simulink model "LIMITATIONS"  (R2024b)
settings: configuration reference "STM32H7_Config" (kept outside this file)
settings Model: DataDictionary=Master_Dictionary.sldd  EnableAccessToBaseWorkspace=off  Creator=torni  LastModifiedBy=William
settings ConfigSetRef: SourceName=STM32H7_Config

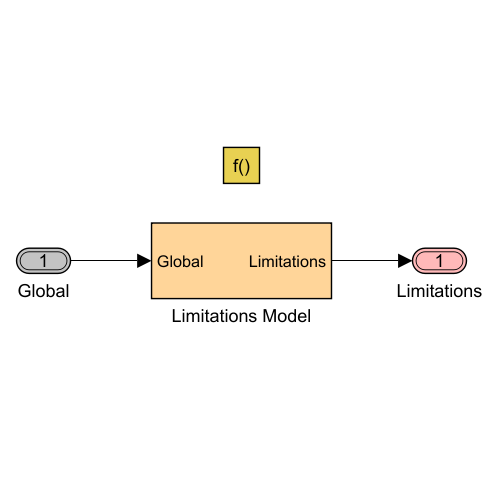
[thumbnail: Simulink's stored preview of the top-level diagram]
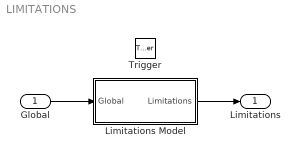
== system LIMITATIONS ==
  "Global " : Inport  OutDataTypeStr=Bus: Global
  Trigger : TriggerPort  TriggerType=function-call  VariantControl=Variant  PortDimensions=1
  "Limitations Model " : Subsystem
  Limitations : Outport  OutDataTypeStr=Bus: LimitationsBus  VectorParamsAs1DForOutWhenUnconnected=off
  wires:
  "Global "/1 -> "Limitations Model "/1(Global)
  "Limitations Model "/1(Limitations) -> Limitations/1

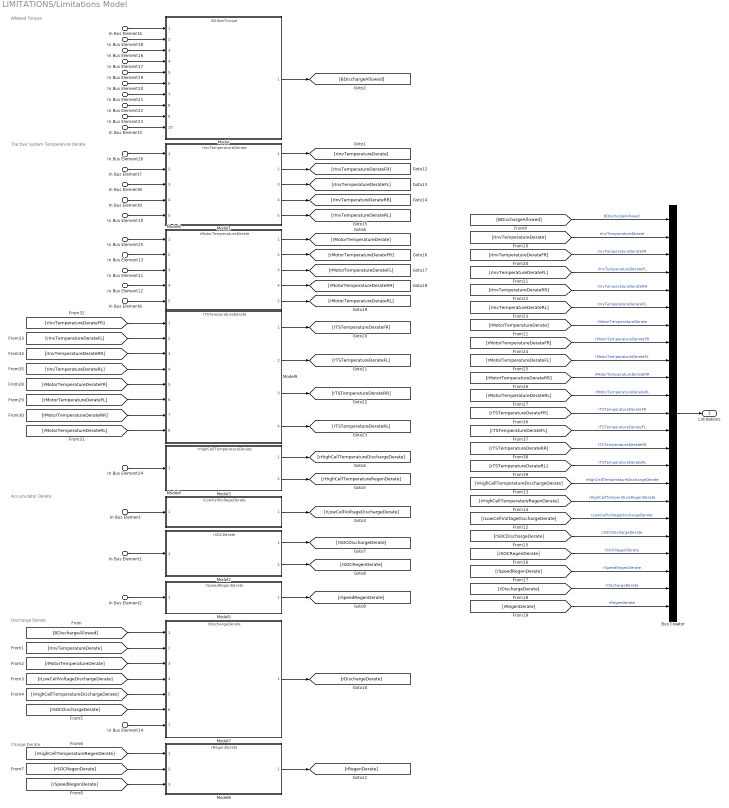
== system LIMITATIONS/Limitations Model  ==
  note: Allowed Torque
  note: Discharge Derate
  note: Charge Derate
  note: Tractive System Temperature Derate
  note: Accumulator Derate
  In Bus Element4 : Inport  PortName=Global  Element=StateflowBus.BReadyToDrive
  In Bus Element16 : Inport  PortName=Global  Element=SystemsBus.BThrottleError
  In Bus Element17 : Inport  PortName=Global  Element=SystemsBus.BBrakeError
  In Bus Element18 : Inport  PortName=Global  Element=SystemsBus.BBrakeOn
  In Bus Element19 : Inport  PortName=Global  Element=SystemsBus.BAppsOK
  In Bus Element25 : Inport  PortName=Global  Element=SystemsBus.TMotorMax
  In Bus Element26 : Inport  PortName=Global  Element=SystemsBus.TInvMax
  In Bus Element2 : Inport  PortName=Global  Element=SystemsBus.vChassis
  In Bus Element14 : Inport  PortName=Global  Element=SystemsBus.BEMSActivated
  In Bus Element20 : Inport  PortName=Global  Element=InverterSignalsBus.InverterFLSignalsBus.nMotorFL
  In Bus Element8 : Inport  PortName=Global  Element=InverterSignalsBus.InverterFLSignalsBus.TInvFL
  In Bus Element11 : Inport  PortName=Global  Element=InverterSignalsBus.InverterFLSignalsBus.TMotorFL
  In Bus Element21 : Inport  PortName=Global  Element=InverterSignalsBus.InverterFRSignalsBus.nMotorFR
  In Bus Element7 : Inport  PortName=Global  Element=InverterSignalsBus.InverterFRSignalsBus.TInvFR
  In Bus Element13 : Inport  PortName=Global  Element=InverterSignalsBus.InverterFRSignalsBus.TMotorFR
  In Bus Element22 : Inport  PortName=Global  Element=InverterSignalsBus.InverterRLSignalsBus.nMotorRL
  In Bus Element10 : Inport  PortName=Global  Element=InverterSignalsBus.InverterRLSignalsBus.TInvRL
  In Bus Element6 : Inport  PortName=Global  Element=InverterSignalsBus.InverterRLSignalsBus.TMotorRL
  In Bus Element23 : Inport  PortName=Global  Element=InverterSignalsBus.InverterRRSignalsBus.nMotorRR
  In Bus Element9 : Inport  PortName=Global  Element=InverterSignalsBus.InverterRRSignalsBus.TInvRR
  In Bus Element12 : Inport  PortName=Global  Element=InverterSignalsBus.InverterRRSignalsBus.TMotorRR
  In Bus Element24 : Inport  PortName=Global  Element=BMSSignalsBus.TCellMax
  In Bus Element : Inport  PortName=Global  Element=BMSSignalsBus.VCellMin
  In Bus Element1 : Inport  PortName=Global  Element=BMSSignalsBus.VDCAccumulator
  In Bus Element3 : Inport  PortName=Global  Element=BMSSignalsBus.IIVTS
  Bus Creator : BusCreator  Inputs=23  OutDataTypeStr=Bus: LimitationsBus
  Model : ModelReference  ModelNameDialog=BAllowTorque  SimulationMode=Normal  ModelReferenceVersion=13.6
  Model1 : ModelReference  ModelNameDialog=rInvTemperatureDerate.slx  SimulationMode=Normal  ModelReferenceVersion=13.6
  Model2 : ModelReference  ModelNameDialog=rSOCDerate.slx  SimulationMode=Normal  ModelReferenceVersion=13.6
  Model3 : ModelReference  ModelNameDialog=rHighCellTemperatureDerate.slx  SimulationMode=Normal  ModelReferenceVersion=13.6
  Model4 : ModelReference  ModelNameDialog=rLowCellVoltageDerate.slx  SimulationMode=Normal  ModelReferenceVersion=13.6
  Model5 : ModelReference  ModelNameDialog=rSpeedRegenDerate.slx  SimulationMode=Normal  ModelReferenceVersion=13.6
  Model6 : ModelReference  ModelNameDialog=rMotorTemperatureDerate.slx  SimulationMode=Normal  ModelReferenceVersion=13.6
  Model7 : ModelReference  ModelNameDialog=rDischargeDerate.slx  SimulationMode=Normal  ModelReferenceVersion=13.5
  Model8 : ModelReference  ModelNameDialog=rRegenDerate.slx  SimulationMode=Normal  ModelReferenceVersion=13.5
  Model9 : ModelReference  ModelNameDialog=rTSTemperatureDerate.slx  SimulationMode=Normal  ModelReferenceVersion=13.5
  Limitations : Outport  OutDataTypeStr=Bus: LimitationsBus  VectorParamsAs1DForOutWhenUnconnected=off
  wires:
  In Bus Element4/1 -> Model/1
  In Bus Element18/1 -> Model/2
  In Bus Element17/1 -> Model/4
  In Bus Element16/1 -> Model/3
  Model/1 -> [BDischargeAllowed]
  In Bus Element26/1 -> Model1/1
  Model1/1 -> [rInvTemperatureDerate]
  Bus Creator/1 -> Limitations/1
  In Bus Element19/1 -> Model/5
  In Bus Element20/1 -> Model/6
  In Bus Element21/1 -> Model/7
  In Bus Element22/1 -> Model/8
  In Bus Element23/1 -> Model/9
  In Bus Element/1 -> Model4/1
  Model4/1 -> [rLowCellVoltageDischargeDerate]
  In Bus Element24/1 -> Model3/1
  Model3/1 -> [rHighCellTemperatureDischargeDerate]
  Model3/2 -> [rHighCellTemperatureRegenDerate]
  In Bus Element25/1 -> Model6/1
  Model6/1 -> [rMotorTemperatureDerate]
  In Bus Element1/1 -> Model2/1
  Model2/1 -> [rSOCDischargeDerate]
  Model2/2 -> [rSOCRegenDerate]
  In Bus Element2/1 -> Model5/1
  Model5/1 -> [rSpeedRegenDerate]
  [rInvTemperatureDerate] -> Model7/2
  [rMotorTemperatureDerate] -> Model7/3
  [rLowCellVoltageDischargeDerate] -> Model7/4
  [rSOCDischargeDerate] -> Model7/6
  [rHighCellTemperatureDischargeDerate] -> Model7/5
  Model7/1 -> [rDischargeDerate]
  [rHighCellTemperatureRegenDerate] -> Model8/1
  [rSOCRegenDerate] -> Model8/2
  [rSpeedRegenDerate] -> Model8/3
  Model8/1 -> [rRegenDerate]
  [BDischargeAllowed] -> Bus Creator/1  "BDischargeAllowed"
  [rInvTemperatureDerate] -> Bus Creator/2  "rInvTemperatureDerate"
  [rMotorTemperatureDerate] -> Bus Creator/7  "rMotorTemperatureDerate"
  [rLowCellVoltageDischargeDerate] -> Bus Creator/18  "rLowCellVoltageDischargeDerate"
  [rHighCellTemperatureDischargeDerate] -> Bus Creator/16  "rHighCellTemperatureDischargeDerate"
  [rHighCellTemperatureRegenDerate] -> Bus Creator/17  "rHighCellTemperatureRegenDerate"
  [rSOCDischargeDerate] -> Bus Creator/19  "rSOCDischargeDerate"
  [rSOCRegenDerate] -> Bus Creator/20  "rSOCRegenDerate"
  [rSpeedRegenDerate] -> Bus Creator/21  "rSpeedRegenDerate"
  [rDischargeDerate] -> Bus Creator/22  "rDischargeDerate"
  [rRegenDerate] -> Bus Creator/23  "rRegenDerate"
  [BDischargeAllowed] -> Model7/1
  In Bus Element3/1 -> Model/10
  Model1/2 -> [rInvTemperatureDerateFR]
  Model1/3 -> [rInvTemperatureDerateFL]
  Model1/4 -> [rInvTemperatureDerateRR]
  Model1/5 -> [rInvTemperatureDerateRL]
  In Bus Element7/1 -> Model1/2
  In Bus Element8/1 -> Model1/3
  In Bus Element9/1 -> Model1/4
  In Bus Element10/1 -> Model1/5
  Model6/2 -> [rMotorTemperatureDerateFR]
  Model6/3 -> [rMotorTemperatureDerateFL]
  Model6/4 -> [rMotorTemperatureDerateRR]
  Model6/5 -> [rMotorTemperatureDerateRL]
  In Bus Element11/1 -> Model6/3
  In Bus Element12/1 -> Model6/4
  In Bus Element6/1 -> Model6/5
  In Bus Element13/1 -> Model6/2
  [rInvTemperatureDerateFR] -> Bus Creator/3  "rInvTemperatureDerateFR"
  [rInvTemperatureDerateRR] -> Bus Creator/5  "rInvTemperatureDerateRR"
  [rInvTemperatureDerateFL] -> Bus Creator/4  "rInvTemperatureDerateFL"
  [rInvTemperatureDerateRL] -> Bus Creator/6  "rInvTemperatureDerateRL"
  [rMotorTemperatureDerateFR] -> Bus Creator/8  "rMotorTemperatureDerateFR"
  [rMotorTemperatureDerateFL] -> Bus Creator/9  "rMotorTemperatureDerateFL"
  [rMotorTemperatureDerateRR] -> Bus Creator/10  "rMotorTemperatureDerateRR"
  [rMotorTemperatureDerateRL] -> Bus Creator/11  "rMotorTemperatureDerateRL"
  In Bus Element14/1 -> Model7/7
  Model9/1 -> [rTSTemperatureDerateFR]
  Model9/2 -> [rTSTemperatureDerateFL]
  Model9/3 -> [rTSTemperatureDerateRR]
  Model9/4 -> [rTSTemperatureDerateRL]
  [rMotorTemperatureDerateFR] -> Model9/5
  [rMotorTemperatureDerateFL] -> Model9/6
  [rMotorTemperatureDerateRR] -> Model9/7
  [rMotorTemperatureDerateRL] -> Model9/8
  [rInvTemperatureDerateFR] -> Model9/1
  [rInvTemperatureDerateFL] -> Model9/2
  [rInvTemperatureDerateRR] -> Model9/3
  [rInvTemperatureDerateRL] -> Model9/4
  [rTSTemperatureDerateFR] -> Bus Creator/12  "rTSTemperatureDerateFR"
  [rTSTemperatureDerateFL] -> Bus Creator/13  "rTSTemperatureDerateFL"
  [rTSTemperatureDerateRR] -> Bus Creator/14  "rTSTemperatureDerateRR"
  [rTSTemperatureDerateRL] -> Bus Creator/15  "rTSTemperatureDerateRL"
